simulink model "Controlpd1"  (R2018a)
settings: Solver=VariableStepAuto  StartTime=0.0  StopTime=10.0  RelTol=1e-3
values from neighbouring files (symbols this model uses):
  kd = 1    [controlpd1.m]
  kd1 = 1    [controlpd1.m]
  kd2 = 1.8    [controlpd1.m]
  kp = 1    [controlpd1.m]
  kp1 = 1    [controlpd1.m]
  kp2 = 4    [controlpd1.m]
settings Model: Creator=ADani  LastModifiedBy=Dell
settings CodeAppCC: StateflowObjectComments=on

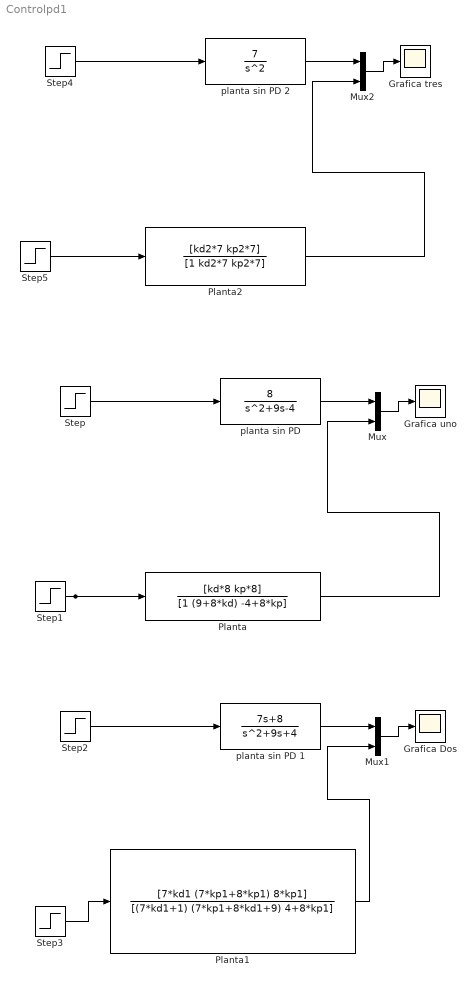
== system Controlpd1 ==
  "Grafica Dos " : Scope
  Grafica tres : Scope
  "Grafica uno " : Scope
  Mux : Mux  Inputs=2
  Mux1 : Mux  Inputs=2
  Mux2 : Mux  Inputs=2
  Planta : TransferFcn  Numerator=[kd*8 kp*8]  Denominator=[1 (9+8*kd) -4+8*kp]
  Planta1 : TransferFcn  Numerator=[7*kd1 (7*kp1+8*kp1) 8*kp1]  Denominator=[(7*kd1+1) (7*kp1+8*kd1+9) 4+8*kp1]
  Planta2 : TransferFcn  Numerator=[kd2*7 kp2*7]  Denominator=[1 kd2*7 kp2*7]
  Step{,1..5} (6 alike) : Step  SampleTime=0
  "planta sin PD " : TransferFcn  Numerator=[8]  Denominator=[1 9 -4]
  planta sin PD 1 : TransferFcn  Numerator=[7 8]  Denominator=[1 9 +4]
  planta sin PD 2 : TransferFcn  Numerator=[7]  Denominator=[1 0 0]
  wires:
  Step/1 -> "planta sin PD "/1
  "planta sin PD "/1 -> Mux/1
  Mux/1 -> "Grafica uno "/1
  Step1/1 -> Planta/1
  Planta/1 -> Mux/2
  Planta1/1 -> Mux1/2
  Step3/1 -> Planta1/1
  Mux1/1 -> "Grafica Dos "/1
  planta sin PD 1/1 -> Mux1/1
  Step2/1 -> planta sin PD 1/1
  Planta2/1 -> Mux2/2
  Step5/1 -> Planta2/1
  Mux2/1 -> Grafica tres/1
  planta sin PD 2/1 -> Mux2/1
  Step4/1 -> planta sin PD 2/1
